simulink model "nuovo_TRACKING"  (R2024b)
settings: Solver=ode4  StartTime=0.0  StopTime=T_SIM  FixedStep=T_s  RelTol=1e-3
values from neighbouring files (symbols this model uses):
  control_par = [k1, k2,b]    [new_traj_tracking_script.m]    (also in traj_tracking_script.m)
  controller_index = 1    [new_traj_tracking_script.m]    (also in traj_tracking_script.m)
  d = d_actual    (= 0.1604)    [new_traj_tracking_script.m]    (also in traj_tracking_script.m)
  D = diag([0.8e-3, 0.8e-3, 5e-3, 0.0175/6, 0.0175/6, 0.0175/6*T_s, 0.0175/6*T_s].^2)    [new_traj_tracking_script.m]    (also in traj_tracking_script.m)
  d_actual = 0.16040    (= 0.1604)    [new_traj_tracking_script.m]    (also in traj_tracking_script.m)
  H_enc = [0, 0, 0, 1, 0, 0, 0 ... (first row only)    [new_traj_tracking_script.m]    (also in traj_tracking_script.m)
  H_gyro = [0, 0, 0, 0, 0, -r_actual/d_actual, r_actual/d_actual]    [new_traj_tracking_script.m]    (also in traj_tracking_script.m)
  H_motion_cap = [1, 0, 0, 0, 0, 0, 0 ... (first row only)    [new_traj_tracking_script.m]    (also in traj_tracking_script.m)
  omega_M = 10    [new_traj_tracking_script.m]    (also in traj_tracking_script.m)
  P_INIT_EKF = diag([0.001, 0.001, 0.0175/6, 0.0175/6, 0.0175/6, 0.0175/6*T_s, 0.0175/6*T_s].^2)    [new_traj_tracking_script.m]    (also in traj_tracking_script.m = diag([0.1, 0.1, 0.1, 0.0175/6, 0.0175/6, 0.0175/6*T_s, 0.017)
  p_loss = p_loss_values(i)    [new_traj_tracking_script.m]    (also in traj_tracking_script.m)
  PHI_INIT = [0;0]    [new_traj_tracking_script.m]    (also in traj_tracking_script.m)
  Q_INIT = [-0.4; -0.5; pi/2]    [new_traj_tracking_script.m]    (also in traj_tracking_script.m)
  Q_INIT_LOC = Q_INIT    [new_traj_tracking_script.m]    (also in traj_tracking_script.m)
  r = r_actual    (= 0.03293)    [new_traj_tracking_script.m]    (also in traj_tracking_script.m)
  R_3 = diag(([sigma_motion_capture, sigma_motion_capture, sigma_motion_capture,               sigma_enc, sigma_enc, sigma_imu]).^2)    [new_traj_tracking_script.m]    (also in traj_tracking_script.m)
  r_actual = 0.03293    [new_traj_tracking_script.m]    (also in traj_tracking_script.m)
  T_s = 0.04    [new_traj_tracking_script.m]    (also in traj_tracking_script.m)
  T_trj = 15    [new_traj_tracking_script.m]    (also in traj_tracking_script.m)
  trj_index = 2    [new_traj_tracking_script.m]    (also in traj_tracking_script.m = 5)
  Z_INIT_EKF = [Q_INIT; 0; 0; 0; 0]    [new_traj_tracking_script.m]    (also in traj_tracking_script.m)
undefined symbols (not defined in the file or in its folder): X, Y
libraries: robotlib x6, sharedtransform x1
(part 2 of 2)

== matlab function nuovo_TRACKING/Localizzazione EKF/MATLAB Function2 ==
  data: P_filt input; P_new output; z_filt input; z_new output; u input; y_new input; D parameter; T_s parameter; r_actual parameter; d_actual parameter; H_enc parameter; H_gyro parameter; H_motion_cap parameter; R_3 parameter; q_EKF output
function [P_new, z_new, q_EKF] = EKF_filtering(P_filt, z_filt, u, y_new, D, T_s, r_actual, d_actual, H_enc, H_gyro, H_motion_cap, R_3)

    % Def state z_filt: [xk , yk , thetak , delta_phi_L_km1 , delta_phi_R_km1 , wLk , wRk ]

    r = r_actual;
    d = d_actual;
        
    % Extraction variables
    x_k = z_filt(1);
    y_k = z_filt(2);
    theta_k = z_filt(3);
    delta_phi_L_km1 = z_filt(4);
    delta_phi_R_km1 = z_filt(5); 
    wL_k = z_filt(6);               % estimate wheels velocities
    wR_k = z_filt(7);
    
    uL_k = u(1);                    % actual wheels velocities (from command input v,w)
    uR_k = u(2);

    % ----------------------

    % PREDICT STEP
    v_k = (r/2) * (wL_k + wR_k);
    omega_k = (r/d) * (wR_k - wL_k);
    theta_mean = theta_k + (omega_k * T_s) / 2;
        
    % State Prediction (approximation with RK2)
    x_kp1 = x_k + v_k * T_s * cos(theta_mean);
    y_kp1 = y_k + v_k * T_s * sin(theta_mean);
    theta_kp1 = theta_k + omega_k * T_s;
    
    delta_phi_L_k = wL_k * T_s;
    delta_phi_R_k = wR_k * T_s;
    
    wL_kp1 = uL_k; 
    wR_kp1 = uR_k;
    
    z_hat = [x_kp1; y_kp1; theta_kp1; delta_phi_L_k; delta_phi_R_k; wL_kp1; wR_kp1];
    
    % F derivation
    F = zeros(7,7);
    
    F(1,1) = 1;
    F(1, 3) = -T_s * v_k * sin(theta_mean);
    F(1, 6) = (T_s * r / 2) * cos(theta_mean) - v_k * T_s * sin(theta_mean) * (-T_s * r / (2 * d));
    F(1, 7) = (T_s * r / 2) * cos(theta_mean) - v_k * T_s * sin(theta_mean) * (T_s * r / (2 * d));
    
    F(2,2) = 1;
    F(2, 3) = v_k * T_s * cos(theta_mean);
    F(2, 6) = (T_s * r / 2) * sin(theta_mean) + v_k * T_s * cos(theta_mean) * (-T_s * r / (2 * d));
    F(2, 7) = (T_s * r / 2) * sin(theta_mean) + v_k * T_s * cos(theta_mean) * (T_s * r / (2 * d));

    F(3,3) = 1;
    F(3, 6) = -T_s * r / d;
    F(3, 7) = T_s * r / d;

    F(4, 6) = T_s;
    F(5, 7) = T_s;
    
    % Covariance Prediction
    P_hat = F * P_filt * F' + D;
    
    % ----------------------

    % UPDATE STEP
    % H and R will depend on the measurement data y_new and Test_case

    % enc_values (delta_phi)
    % IMU_values (w_gyro)
    % Motion_capture (state q)

    % y_new = [x; y; theta; delta_phi_L; delta_phi_R; omega_gyro]

    %% OBSERVATION MATRIX H ALWAYS FULL (6X7) AND ALSO Y_NEW (6X1) 
    H_full = [H_motion_cap; H_enc; H_gyro];
    y_meas = y_new; 
    
    % Start with full matrix R_3 
    R_current = R_3;
    INFINITY_VAR = 1e9; % Infinite var to put down the Kalman gain
    
    % IMU not available
    R_current(6,6) = INFINITY_VAR; 

    % TEST 3: all active, possibile data loss
    if any(isnan(y_new(1:3)))   
        y_meas(1:3) = 0;    % force to zero just for completness
        R_current(1,1) = INFINITY_VAR; 
        R_current(2,2) = INFINITY_VAR; 
        R_current(3,3) = INFINITY_VAR;
    end

    
    % Innovation e_pred
    y_hat = H_full * z_hat;
    e_kp1 = y_meas - y_hat;
    
    % Kalman Gain K_pred
    K = P_hat * H_full' / (H_full * P_hat * H_full' + R_current);   
    
    % State and Covariance Update
    z_new = z_hat + K * e_kp1;
    P_new = P_hat - K * H_full * P_hat;

    q_EKF = z_new(1:3);


end

== matlab function nuovo_TRACKING/Norm cartesian error ==
  data: u input; y output
function y = fcn(u)

y = sqrt(sum(u(1:2).^2));

== matlab function nuovo_TRACKING/Norm error ==
  data: u input; y output
function y = fcn(u)
y = [u(1);u(2); wrapToPi(u(3))];
